simulink model "RecordEEG"  (R2020b)
settings: Solver=FixedStepAuto  StartTime=0.0  StopTime=inf  RelTol=1e-3  EnableMultiTasking=on
libraries: simulink x2, arduinolib x1
settings Model: SimulationMode=external  SILPILModeSetting=veronly  EnablePacing=on  ExtModeTrigDuration=2  Creator=plaserst  LastModifiedBy=plaserst
settings OptimizationCC: EnhancedBackFolding=on  PassReuseOutputArgsAs=Individual arguments  ZeroExternalMemoryAtStartup=off  ZeroInternalMemoryAtStartup=off  MaxStackSize=64  OptimizeBlockOrder=speed  DifferentSizesBufferReuse=on  OptimizationCustomize=off  EfficientTunableParamExpr=on
settings DebuggingCC: ParameterTunabilityLossMsg=error
settings HardwareCC: ProdBitPerInt=16  ProdBitPerPointer=16  ProdBitPerSizeT=16  ProdBitPerPtrDiffT=16  ProdLargestAtomicFloat=None  ProdWordSize=8  ProdHWDeviceType=Atmel->AVR
settings SFSimCC: MATLABDynamicMemAlloc=off
settings RTWCC: Description=Embedded Coder  SystemTargetFile=ert.tlc  HardwareBoard=Arduino Uno  TemplateMakefile=ert_default_tmf  Toolchain=Arduino AVR  BuildConfiguration=Faster Runs
settings CodeAppCC: ForceParamTrailComments=on  IgnoreCustomStorageClasses=off  OperatorAnnotations=on  SimulinkDataObjDesc=on  SFDataObjDesc=on  InsertBlockDesc=on
settings ERTTargetCC: SupportContinuousTime=on  SupportVariableSizeSignals=on  ExtModeStaticAllocSize=250

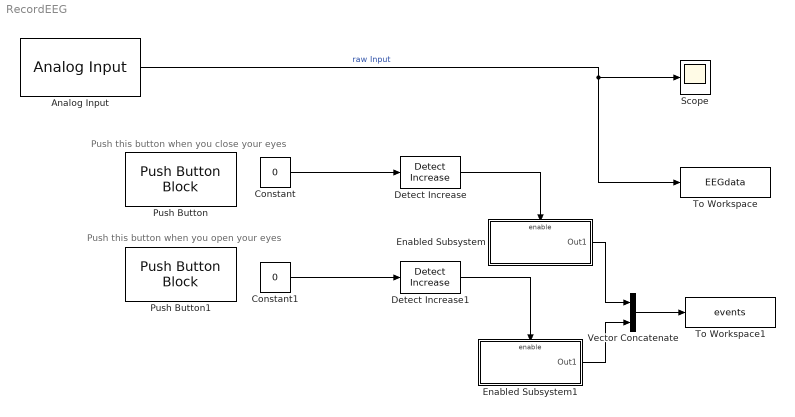
== system RecordEEG ==
  note: Push this button when you close your eyes
  note: Push this button when you open your eyes
  Analog Input : arduinolib/Analog Input  pinNumber=0  ReadResultsOnly=off  ConversionTriggerSource=Software  ExternalTriggerType=uint32( 0 )  OutputDataType=uint16  EnableConversionCompleteNotify=off  EnableOuputStatus=off  SampleTime=1/250  blockPlatform=arduino
  Constant : Constant  Value=0  SampleTime=-1
  Constant1 : Constant  Value=0  SampleTime=-1
  Detect Increase : simulink/Logic and Bit Operations/Detect Increase  vinit=0.0  OutDataTypeStr=boolean
  Detect Increase1 : simulink/Logic and Bit Operations/Detect Increase  vinit=0.0  OutDataTypeStr=boolean
  Enabled Subsystem : Subsystem  TreatAsAtomicUnit=on
  Enabled Subsystem1 : Subsystem  TreatAsAtomicUnit=on
  Push Button : PushButtonBlock  ButtonText=Eyes closed
  Push Button1 : PushButtonBlock  ButtonText=Eyes opened
  Scope : Scope
  To Workspace : ToWorkspace  VariableName=EEGdata  SaveFormat=Structure With Time  SampleTime=-1
  To Workspace1 : ToWorkspace  VariableName=events  SaveFormat=Timeseries  SampleTime=-1
  Vector Concatenate : Concatenate
  wires:
  Analog Input/1 -> Scope/1, To Workspace/1  "raw Input"
  Enabled Subsystem/1(Out1) -> Vector Concatenate/1
  Constant/1 -> Detect Increase/1
  Constant1/1 -> Detect Increase1/1
  Enabled Subsystem1/1(Out1) -> Vector Concatenate/2
  Vector Concatenate/1 -> To Workspace1/1
  Detect Increase/1 -> Enabled Subsystem/Enable
  Detect Increase1/1 -> Enabled Subsystem1/Enable

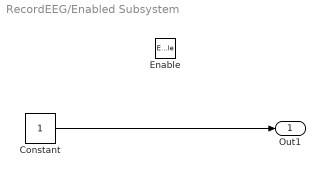
== system RecordEEG/Enabled Subsystem ==
  Enable : EnablePort
  Constant : Constant  SampleTime=-1
  Out1 : Outport  OutputWhenDisabled=reset  InitialOutput=0
  wires:
  Constant/1 -> Out1/1

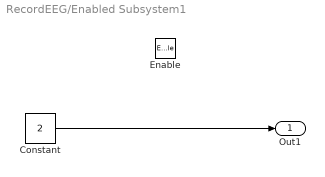
== system RecordEEG/Enabled Subsystem1 ==
  Enable : EnablePort
  Constant : Constant  Value=2  SampleTime=-1
  Out1 : Outport  OutputWhenDisabled=reset  InitialOutput=0
  wires:
  Constant/1 -> Out1/1
